simulink model "system_model"  (R2020b)
settings: Solver=VariableStepAuto  StartTime=0.0  StopTime=10.0  RelTol=1e-3
values from neighbouring files (symbols this model uses):
  b = 20    [system_init.m]
  k1 = 50    [system_init.m]
  k2 = 60    [system_init.m]
  m1 = 500    [system_init.m]
  m2 = 20    [system_init.m]
settings Model: Creator=Admin  LastModifiedBy=Admin

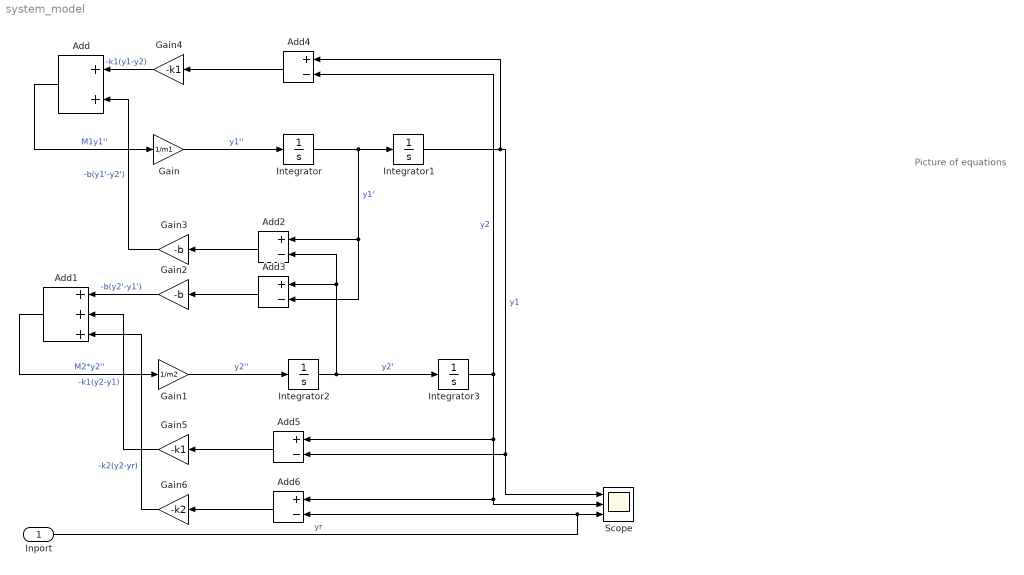
== system system_model ==
  note: Picture of equations
  Inport : Inport
  Add : Sum
  Add1 : Sum  Inputs=+++
  Add{2..6} (5 alike) : Sum  Inputs=+-
  Gain : Gain  Gain=1/m1
  Gain1 : Gain  Gain=1/m2
  Gain2 : Gain  Gain=-b
  Gain3 : Gain  Gain=-b
  Gain4 : Gain  Gain=-k1
  Gain5 : Gain  Gain=-k1
  Gain6 : Gain  Gain=-k2
  Integrator{,1..3} (4 alike) : Integrator
  Scope : Scope  NumInputPorts=3
  wires:
  Gain4/1 -> Add/1  "-k1(y1-y2)"
  Gain3/1 -> Add/2  "-b(y1'-y2')"
  Integrator1/1 -> Add5/2, Scope/1, Add4/1  "y1"
  Gain2/1 -> Add1/1  "-b(y2'-y1')"
  Add2/1 -> Gain3/1
  Integrator2/1 -> Integrator3/1, Add3/1, Add2/2  "y2'"
  Gain1/1 -> Integrator2/1  "y2''"
  Add5/1 -> Gain5/1
  Add3/1 -> Gain2/1
  Add6/1 -> Gain6/1
  Gain6/1 -> Add1/3  "-k2(y2-yr)"
  Add/1 -> Gain/1  "M1y1''"
  Gain/1 -> Integrator/1  "y1''"
  Inport/1 -> Scope/3, Add6/2  "yr"
  Integrator/1 -> Add3/2, Add2/1, Integrator1/1  "y1'"
  Integrator3/1 -> Scope/2, Add6/1, Add5/1, Add4/2  "y2"
  Gain5/1 -> Add1/2  "-k1(y2-y1)"
  Add1/1 -> Gain1/1  "M2*y2''"
  Add4/1 -> Gain4/1
